simulink model "BodyHalf_Verif"  (R2021b)
settings: Solver=VariableStepAuto  StartTime=0.0  StopTime=10.0  RelTol=1e-3
values from neighbouring files (symbols this model uses):
  a = b    (= 1.4)    [CarQuarterParam.m]
  b = 1.4    [CarQuarterParam.m]
  I = 600    [CarQuarterParam.m]
  M1 = 500    [CarQuarterParam.m]
settings Model: Creator=Reece Bell  LastModifiedBy=reece
settings SolverCC: AlgebraicLoopSolver=TrustRegion
settings DataIOCC: ReturnWorkspaceOutputs=off
settings DebuggingCC: SFMachineParentedDataDiag=warning  ArithmeticOperatorsInVariantConditions=warning
settings SFSimCC: CustomCodeUndefinedFunction=UseInterfaceOnly

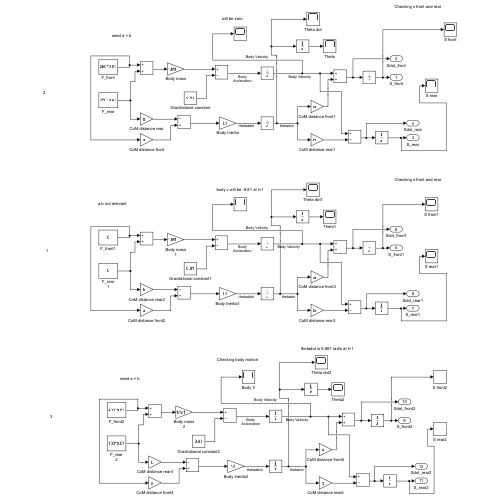
[thumbnail: Simulink's stored preview of the top-level diagram]
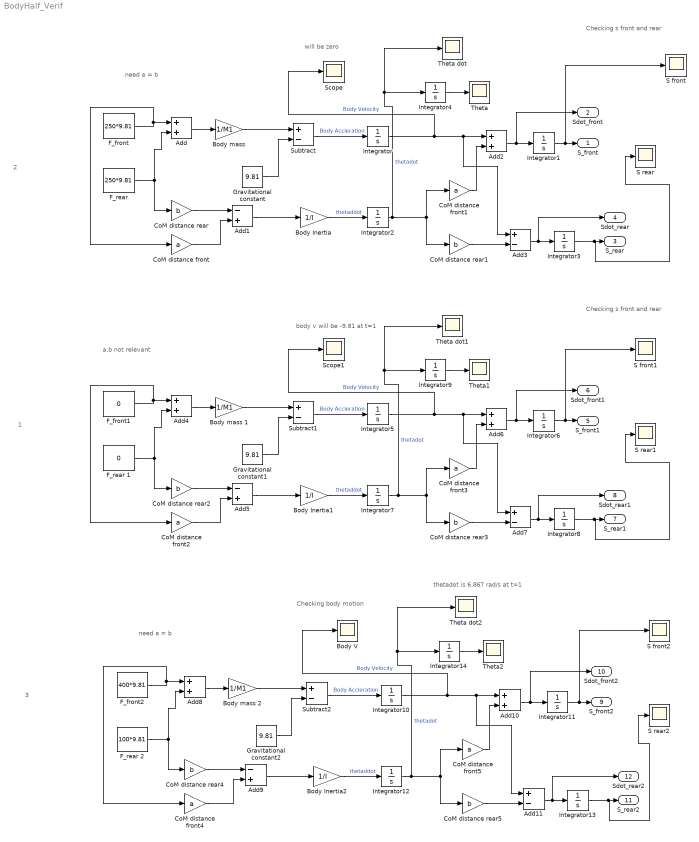
== system BodyHalf_Verif ==
  note: 3
  note: 2
  note: 1
  note: will be zero
  note: body v will be -9.81 at t=1
  note: thetadot is 6.867 rad/s at t=1
  note: Checking body motion
  note: Checking s front and rear
  note: a,b not relevant
  note: need a = b
  note: need a = b
  note: Checking s front and rear
  Add{,2,4,6,8,10} (6 alike) : Sum
  Add1 : Sum  Inputs=-+
  Add11 : Sum  Inputs=+-
  Add3 : Sum  Inputs=+-
  Add5 : Sum  Inputs=-+
  Add7 : Sum  Inputs=+-
  Add9 : Sum  Inputs=-+
  Body Inertia : Gain  Gain=1/I
  Body Inertia1 : Gain  Gain=1/I
  Body Inertia2 : Gain  Gain=1/I
  Body V : Scope
  "Body mass " : Gain  Gain=1/M1
  Body mass 1 : Gain  Gain=1/M1
  Body mass 2 : Gain  Gain=1/M1
  CoM distance front{,1..5} (6 alike) : Gain  Gain=a
  CoM distance rear{,1..5} (6 alike) : Gain  Gain=b
  F_front : Constant  Value=250*9.81
  F_front1 : Constant  Value=0
  F_front2 : Constant  Value=400*9.81
  "F_rear " : Constant  Value=250*9.81
  F_rear 1 : Constant  Value=0
  F_rear 2 : Constant  Value=100*9.81
  Gravitational constant : Constant  Value=9.81
  Gravitational constant1 : Constant  Value=9.81
  Gravitational constant2 : Constant  Value=9.81
  Integrator{,1..14} (15 alike) : Integrator
  S front : Scope
  S front1 : Scope
  S front2 : Scope
  S rear : Scope
  S rear1 : Scope
  S rear2 : Scope
  Scope : Scope
  Scope1 : Scope
  Subtract : Sum  Inputs=+-
  Subtract1 : Sum  Inputs=+-
  Subtract2 : Sum  Inputs=+-
  Theta : Scope
  Theta dot : Scope
  Theta dot1 : Scope
  Theta dot2 : Scope
  Theta1 : Scope
  Theta2 : Scope
  S_front : Outport  VectorParamsAs1DForOutWhenUnconnected=off
  Sdot_front : Outport  Port=2  VectorParamsAs1DForOutWhenUnconnected=off
  S_rear : Outport  Port=3  VectorParamsAs1DForOutWhenUnconnected=off
  Sdot_rear : Outport  Port=4  VectorParamsAs1DForOutWhenUnconnected=off
  S_front1 : Outport  Port=5  VectorParamsAs1DForOutWhenUnconnected=off
  Sdot_front1 : Outport  Port=6  VectorParamsAs1DForOutWhenUnconnected=off
  S_rear1 : Outport  Port=7  VectorParamsAs1DForOutWhenUnconnected=off
  Sdot_rear1 : Outport  Port=8  VectorParamsAs1DForOutWhenUnconnected=off
  S_front2 : Outport  Port=9  VectorParamsAs1DForOutWhenUnconnected=off
  Sdot_front2 : Outport  Port=10  VectorParamsAs1DForOutWhenUnconnected=off
  S_rear2 : Outport  Port=11  VectorParamsAs1DForOutWhenUnconnected=off
  Sdot_rear2 : Outport  Port=12  VectorParamsAs1DForOutWhenUnconnected=off
  wires:
  Add3/1 -> Sdot_rear/1, Integrator3/1
  Body Inertia/1 -> Integrator2/1  "thetaddot"
  Gravitational constant/1 -> Subtract/2
  Integrator/1 -> Scope/1, Add3/1, Add2/1  "Body Velocity"
  Integrator2/1 -> CoM distance rear1/1, CoM distance front1/1, Integrator4/1, Theta dot/1  "thetadot"
  Add2/1 -> Sdot_front/1, Integrator1/1
  CoM distance rear/1 -> Add1/1
  Add/1 -> "Body mass "/1
  CoM distance rear1/1 -> Add3/2
  CoM distance front/1 -> Add1/2
  Add1/1 -> Body Inertia/1
  Subtract/1 -> Integrator/1  "Body Accleration"
  "Body mass "/1 -> Subtract/1
  F_front/1 -> Add/1, CoM distance front/1
  CoM distance front1/1 -> Add2/2
  "F_rear "/1 -> Add/2, CoM distance rear/1
  Integrator4/1 -> Theta/1
  Integrator1/1 -> S front/1, S_front/1
  Integrator3/1 -> S rear/1, S_rear/1
  Add5/1 -> Body Inertia1/1
  CoM distance rear3/1 -> Add7/2
  Add4/1 -> Body mass 1/1
  CoM distance front2/1 -> Add5/2
  Subtract1/1 -> Integrator5/1  "Body Accleration"
  F_front1/1 -> Add4/1, CoM distance front2/1
  Add6/1 -> Sdot_front1/1, Integrator6/1
  CoM distance rear2/1 -> Add5/1
  Body Inertia1/1 -> Integrator7/1  "thetaddot"
  Gravitational constant1/1 -> Subtract1/2
  Integrator5/1 -> Scope1/1, Add7/1, Add6/1  "Body Velocity"
  Add7/1 -> Sdot_rear1/1, Integrator8/1
  Integrator7/1 -> Integrator9/1, Theta dot1/1, CoM distance rear3/1, CoM distance front3/1  "thetadot"
  Body mass 1/1 -> Subtract1/1
  Integrator6/1 -> S front1/1, S_front1/1
  Integrator8/1 -> S rear1/1, S_rear1/1
  F_rear 1/1 -> Add4/2, CoM distance rear2/1
  Integrator9/1 -> Theta1/1
  CoM distance front3/1 -> Add6/2
  Add9/1 -> Body Inertia2/1
  CoM distance rear5/1 -> Add11/2
  Add8/1 -> Body mass 2/1
  CoM distance front4/1 -> Add9/2
  Subtract2/1 -> Integrator10/1  "Body Accleration"
  F_front2/1 -> Add8/1, CoM distance front4/1
  Add10/1 -> Sdot_front2/1, Integrator11/1
  CoM distance rear4/1 -> Add9/1
  Body Inertia2/1 -> Integrator12/1  "thetaddot"
  Gravitational constant2/1 -> Subtract2/2
  Integrator10/1 -> Body V/1, Add11/1, Add10/1  "Body Velocity"
  Add11/1 -> Sdot_rear2/1, Integrator13/1
  Integrator12/1 -> Integrator14/1, Theta dot2/1, CoM distance rear5/1, CoM distance front5/1  "thetadot"
  Body mass 2/1 -> Subtract2/1
  Integrator11/1 -> S front2/1, S_front2/1
  Integrator13/1 -> S rear2/1, S_rear2/1
  F_rear 2/1 -> Add8/2, CoM distance rear4/1
  Integrator14/1 -> Theta2/1
  CoM distance front5/1 -> Add10/2
